simulink model "cm_gap_model"  (Simulink 9.3)
settings: Solver=ode23s  StartTime=0.0  StopTime=1  EnableMultiTasking=on
values from neighbouring files (symbols this model uses):
  fase = 0    [sim_cm_gap.m]
  V1 = sqrt(2)*120    [sim_cm_gap.m]    (also in sim_cm_sat.m)
  wb = 2*pi*F    (= 376.991118431)    [cm_init.m]    (also in sim_cm_gap.m)
settings Model: Creator=Alberto  LastModifiedBy=asanchez
settings DataIOCC: LimitDataPoints=on  SignalLoggingName=sigsOut
settings OptimizationCC: ExpressionDepthLimit=2147483647
settings DebuggingCC: AlgebraicLoopMsg=none  SaveWithParameterizedLinksMsg=none  SignalResolutionControl=TryResolveAllWithWarning  MultiTaskDSMMsg=warning  MultiTaskCondExecSysMsg=none  StateNameClashWarn=warning
settings HardwareCC: TargetUnknown=on
settings GRTTargetCC: GeneratePreprocessorConditionals=Disable all

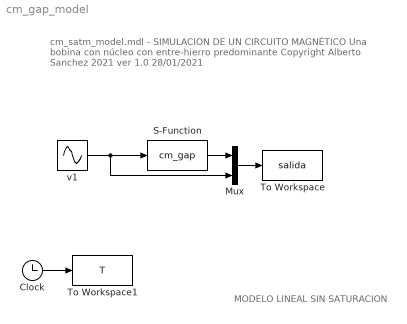
== system cm_gap_model ==
  note: MODELO LINEAL SIN SATURACION
  note: cm_satm_model.mdl - SIMULACION DE UN CIRCUITO MAGNÉTICO
      | Una bobina con núcleo con entre-hierro predominante
      | Copyright Alberto Sanchez 2021
      | ver 1.0 28/01/2021
  Clock : Clock
  Mux : Mux  Inputs=2
  S-Function : S-Function  FunctionName=cm_gap  Parameters=XINIT PAR  SFunctionDeploymentMode=off  EnableBusSupport=off
  To Workspace : ToWorkspace  VariableName=salida  SampleTime=-1
  To Workspace1 : ToWorkspace  VariableName=T  SampleTime=-1
  v1 : Sin  Amplitude=V1  Frequency=wb  Phase=fase  SampleTime=0
  wires:
  v1/1 -> Mux/2, S-Function/1
  Clock/1 -> To Workspace1/1
  Mux/1 -> To Workspace/1
  S-Function/1 -> Mux/1
